simulink model "statemodel"  (Simulink 3.00)
settings: Solver=ode45  SolverMode=SingleTasking  StartTime=0.0  StopTime=10.0  RelTol=1e-3  AbsTol=1e-6
undefined symbols (not defined in the file): C, L, R
settings Model: LastModifiedBy=eechris

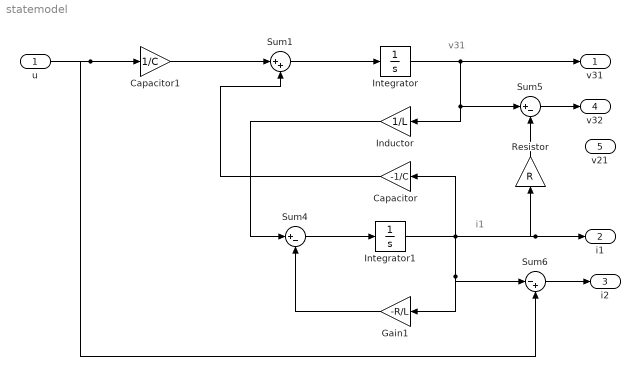
== system statemodel ==
  note: v31
  note: i1
  u : Inport  Port=1  PortWidth=-1  SampleTime=-1  DataType=auto
      settings: SignalType=auto
  Capacitor : Gain  Orientation=left  Gain=-1/C  SaturateOnIntegerOverflow=on
  Capacitor1 : Gain  Gain=1/C  SaturateOnIntegerOverflow=on
  Gain1 : Gain  Orientation=left  Gain=-R/L  SaturateOnIntegerOverflow=on
  Inductor : Gain  Orientation=left  Gain=1/L  SaturateOnIntegerOverflow=on
  Integrator : Integrator  ExternalReset=none  InitialConditionSource=internal  InitialCondition=0  LimitOutput=off  UpperSaturationLimit=inf  LowerSaturationLimit=-inf  ShowSaturationPort=off  ShowStatePort=off  AbsoluteTolerance=auto
  Integrator1 : Integrator  ExternalReset=none  InitialConditionSource=internal  InitialCondition=0  LimitOutput=off  UpperSaturationLimit=inf  LowerSaturationLimit=-inf  ShowSaturationPort=off  ShowStatePort=off  AbsoluteTolerance=auto
  Resistor : Gain  Orientation=up  Gain=R  SaturateOnIntegerOverflow=on
  Sum1 : Sum  Inputs=|++  SaturateOnIntegerOverflow=on
  Sum4 : Sum  Inputs=|+-  SaturateOnIntegerOverflow=on
  Sum5 : Sum  Inputs=|+-  SaturateOnIntegerOverflow=on
  Sum6 : Sum  Inputs=|-+  SaturateOnIntegerOverflow=on
  v31 : Outport  Port=1
  i1 : Outport  Port=2
  i2 : Outport  Port=3
  v32 : Outport  Port=4
  v21 : Outport  Port=5
  wires:
  Sum4/1 -> Integrator1/1
  Integrator1/1 -> Capacitor/1, i1/1, Resistor/1, Gain1/1, Sum6/1
  Capacitor/1 -> Sum1/2
  Sum1/1 -> Integrator/1
  Integrator/1 -> v31/1, Inductor/1, Sum5/1
  Sum6/1 -> i2/1
  Sum5/1 -> v32/1
  Capacitor1/1 -> Sum1/1
  Gain1/1 -> Sum4/2
  Inductor/1 -> Sum4/1
  Resistor/1 -> Sum5/2
  u/1 -> Capacitor1/1, Sum6/2
